simulink model "vertical"  (R2021a)
settings: Solver=VariableStepAuto  StartTime=0.0  StopTime=10.0  RelTol=1e-3
values from neighbouring files (symbols this model uses):
  cu1 = 1    [verticalParameters.m]
  cu2 = 1    [verticalParameters.m]
  Jms = 0.5    [verticalParameters.m]
  ko1 = 1    [verticalParameters.m]
  ku1 = 1    [verticalParameters.m]
  ku2 = 1    [verticalParameters.m]
  ls1 = 0.8    [verticalParameters.m]
  ls2 = 0.8    [verticalParameters.m]
  Ms = 5    [verticalParameters.m]
  Mu1 = 1    [verticalParameters.m]
  Mu2 = 1    [verticalParameters.m]
settings Model: Creator=danie  LastModifiedBy=danie

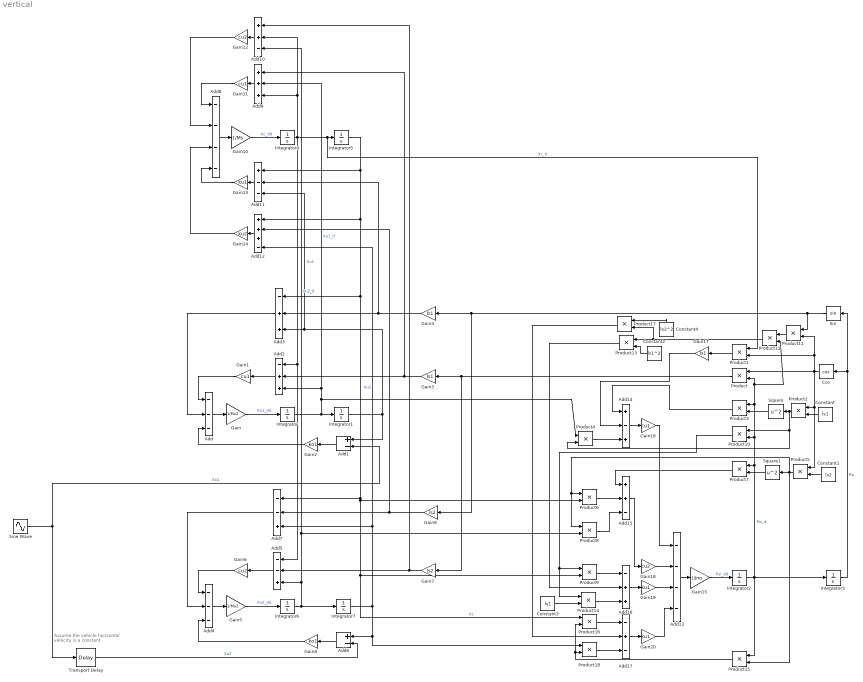
== system vertical ==
  note: Assume the vehicle horizontal velocity is a constant
  Add : Sum  Inputs=---
  Add1 : Sum  Inputs=+-
  Add10 : Sum  Inputs=++-
  Add11 : Sum  Inputs=+--
  Add12 : Sum  Inputs=+++-
  Add13 : Sum  Inputs=----
  Add14 : Sum  Inputs=+-+
  Add15 : Sum  Inputs=++-
  Add16 : Sum  Inputs=-++
  Add17 : Sum  Inputs=-+-
  Add2 : Sum  Inputs=-++
  Add3 : Sum  Inputs=-++
  Add4 : Sum  Inputs=---
  Add5 : Sum  Inputs=--+
  Add6 : Sum  Inputs=+-
  Add7 : Sum  Inputs=--+
  Add8 : Sum  Inputs=----
  Add9 : Sum  Inputs=+++
  Constant : Constant  Value=ls1
  Constant1 : Constant  Value=ls2
  Constant2 : Constant  Value=ls1^2
  Constant3 : Constant  Value=ls1
  Constant4 : Constant  Value=ls2^2
  Cos : Trigonometry  Operator=cos
  Gain : Gain  Gain=1/Mu1
  Gain1 : Gain  Gain=cu1
  Gain10 : Gain  Gain=1/Ms
  Gain11 : Gain  Gain=cu1
  Gain12 : Gain  Gain=cu2
  Gain13 : Gain  Gain=ku1
  Gain14 : Gain  Gain=ku2
  Gain15 : Gain  Gain=1/Jms
  Gain16 : Gain  Gain=cu1
  Gain17 : Gain  Gain=ls1
  Gain18 : Gain  Gain=cu2
  Gain19 : Gain  Gain=ku1
  Gain2 : Gain  Gain=ko1
  Gain20 : Gain  Gain=ku1
  Gain3 : Gain  Gain=ls1
  Gain4 : Gain  Gain=ls1
  Gain5 : Gain  Gain=1/Mu2
  Gain6 : Gain  Gain=cu2
  Gain7 : Gain  Gain=ls2
  Gain8 : Gain  Gain=ko1
  Gain9 : Gain  Gain=ls2
  Integrator{,1..7} (8 alike) : Integrator
  Product{,1..18} (19 alike) : Product
  Sin : Trigonometry
  Sine Wave : Sin  SampleTime=0
  Square : Math  Operator=square  SaturateOnIntegerOverflow=on
  Square1 : Math  Operator=square  SaturateOnIntegerOverflow=on
  Transport Delay : TransportDelay
  wires:
  Gain/1 -> Integrator/1  "Xu1_dd"
  Integrator/1 -> Integrator1/1, Product4/1, Add9/2, Add2/3  "Xu1_d"
  Integrator1/1 -> Add11/3, Add3/3, Add1/1  "Xu1"
  Gain15/1 -> Integrator2/1  "Psi_dd"
  Integrator2/1 -> Product15/1, Integrator3/1, Product10/2, Product12/2, Product/2, Product3/1, Product7/1  "Psi_d"
  Add/1 -> Gain/1
  Integrator4/1 -> Add9/3, Add10/2, Product1/1, Integrator5/1, Add5/1, Add2/1  "Xc_d"
  Gain10/1 -> Integrator4/1  "Xc_dd"
  Integrator5/1 -> Product16/1, Product9/2, Product6/2, Add7/1, Add3/1, Add12/1, Add11/1  "Xc"
  Gain1/1 -> Add/1
  Sine Wave/1 -> Add1/2, Transport Delay/1  "Xo1"
  Add1/1 -> Gain2/1
  Gain2/1 -> Add/3
  Add2/1 -> Gain1/1
  Integrator3/1 -> Sin/1, Cos/1  "Psi"
  Cos/1 -> Product/1, Product11/2, Product1/2, Product2/1, Product5/1
  Product/1 -> Gain7/1, Gain3/1
  Gain3/1 -> Add9/1, Add2/2
  Sin/1 -> Product11/1, Gain9/1, Gain4/1
  Gain4/1 -> Add11/2, Add3/2
  Add3/1 -> Add/2
  Integrator6/1 -> Integrator7/1, Product8/2, Add10/3, Add5/3  "Xu2_d"
  Gain5/1 -> Integrator6/1  "Xu2_dd"
  Add4/1 -> Gain5/1
  Integrator7/1 -> Add12/4, Add7/3, Add6/1, Product18/1  "Xu2"
  Add5/1 -> Gain6/1
  Gain6/1 -> Add4/1
  Gain7/1 -> Add10/1, Add5/2
  Add6/1 -> Gain8/1
  Transport Delay/1 -> Add6/2  "Xo2"
  Gain8/1 -> Add4/3
  Gain9/1 -> Add12/2, Add7/2
  Add7/1 -> Add4/2
  Add8/1 -> Gain10/1
  Add9/1 -> Gain11/1
  Gain11/1 -> Add8/1
  Add10/1 -> Gain12/1
  Gain12/1 -> Add8/2
  Add11/1 -> Gain13/1
  Gain13/1 -> Add8/4
  Add12/1 -> Gain14/1
  Gain14/1 -> Add8/3
  Add13/1 -> Gain15/1
  Gain16/1 -> Add13/1
  Add14/1 -> Gain16/1
  Product1/1 -> Gain17/1
  Gain17/1 -> Add14/2
  Constant/1 -> Product2/2
  Product2/1 -> Product10/1, Product4/2, Square/1
  Square/1 -> Product3/2
  Product3/1 -> Add14/1
  Product4/1 -> Add14/3
  Add15/1 -> Gain18/1
  Gain18/1 -> Add13/2
  Constant1/1 -> Product5/2
  Product6/1 -> Add15/2
  Product5/1 -> Product15/2, Square1/1, Product8/1, Product6/1
  Square1/1 -> Product7/2
  Product7/1 -> Add15/1
  Product8/1 -> Add15/3
  Add16/1 -> Gain19/1
  Gain19/1 -> Add13/3
  Product9/1 -> Add16/1
  Product10/1 -> Product14/1, Product9/1
  Product11/1 -> Product12/1
  Product12/1 -> Product17/2, Product13/1
  Constant2/1 -> Product13/2
  Product13/1 -> Add16/2
  Constant3/1 -> Product14/2
  Product14/1 -> Add16/3
  Add17/1 -> Gain20/1
  Gain20/1 -> Add13/4
  Product16/1 -> Add17/1
  Product15/1 -> Product16/2, Product18/2
  Constant4/1 -> Product17/1
  Product17/1 -> Add17/2
  Product18/1 -> Add17/3
